simulink model "planta_CODESYS"  (R2025b)
settings: Solver=FixedStepAuto  StartTime=0.0  StopTime=inf  FixedStep=Ts2  MaxStep=1e-3  RelTol=1e-3
undefined symbols (not defined in the file): ah_max, at_max, bcx, bcy, bh_eq, bhb, bhEb, bhwu, bt, bt_eq, btb, btw, g, Hc, ih, it, Jh_eq, Jt_eq, Kcy, khwu, Ki_h, Ki_t, Kp_h, Kp_t, Ktw, lambda, Lh, Lh0, lh_0, Lt, magnitude, Mc_max, Ms, Mt, rhd, rtd, tau_hm, tau_tm, Thb_Max, ThEb_Max, Thm_0, Thm_Max, titahm_0, titatm_0, Ts0, Ts1, Ts2, Ttb_Max, Ttm_0, Ttm_Max, vh_0, vlx_0, vly_0, vt_0, vt_max, Wc, whm_0, whm_rated, wtm_0, xl_0 ... (+9)
libraries: simulink x10, opcualib x9, simulink_extras x2, dspnetwork x2, sl3dlib x1, hostiolib x1
(part 1 of 2)
settings Model: Creator=Nahuel  LastModifiedBy=nahue
settings SolverCC: ZeroCrossControl=DisableAll
settings DebuggingCC: UnderSpecifiedDimensionMsg=warning
settings SFSimCC: SimTargetLang=C++  SimDLTargetLibrary=mkl-dnn
settings RTWCC: GPUComputeCapability=3.5

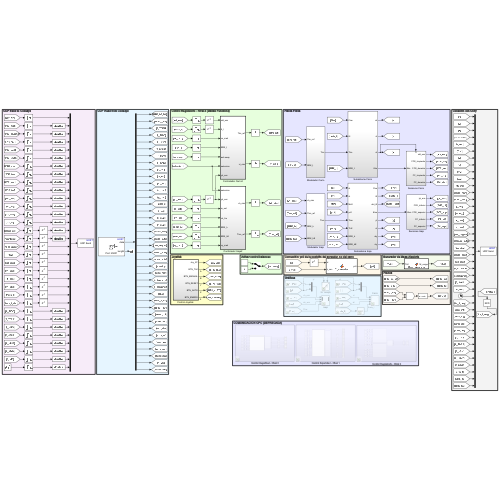
[thumbnail: Simulink's stored preview of the top-level diagram]
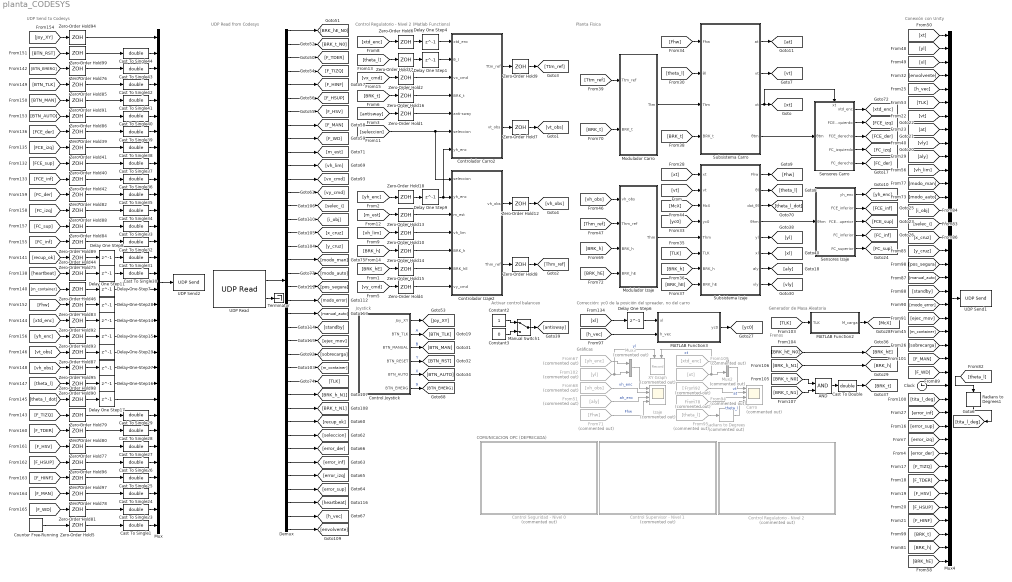
== system planta_CODESYS ==
  note: COMUNICACION OPC (DEPRECADA)
  note: UDP Read from Codesys
  note: UDP Send to Codesys
  note: Joystick
  note: Conexión con Unity
  note: Planta Física
  note: Control Regulatorio - Nivel 2 (Matlab Functions)
  note: Generador de Masa Aleatoria
  note: Corrección: yc0 de la posición del spreader, no del carro
  note: Activar control balanceo
  note: Frenos
  note: Gráficas
  AND : Logic  IconShape=distinctive  AllPortsSameDT=off  OutDataTypeStr=boolean
  Carro : Scope  Commented=on  NumInputPorts=4
      settings: AxesScalingNumUpdates=5  ActiveDisplayYMinimum=-26.90845  ActiveDisplayYMaximum=42.17601
  Cast To Double : DataTypeConversion  OutDataTypeStr=double  SaturateOnIntegerOverflow=off  RndMeth=Floor
  Cast To Single{1,23..44} (23 alike) : DataTypeConversion  OutDataTypeStr=double  SaturateOnIntegerOverflow=off  RndMeth=Floor
  Clock : Clock
  Constant2 : Constant
  Constant3 : Constant  Value=0
  "Control Joystick " : Subsystem  TreatAsAtomicUnit=on  SystemSampleTime=Ts2
  "Control Regulatorio - Nivel 2 " : Subsystem  Commented=on
  Control Seguridad - Nivel 0 : Subsystem  Commented=on
  Control Supervisor - Nivel 1 : Subsystem  Commented=on
  Controlador Carro2 : Subsystem  Priority=3  TreatAsAtomicUnit=on  SystemSampleTime=Ts2
  Controlador Izaje2 : Subsystem  Priority=3  TreatAsAtomicUnit=on  SystemSampleTime=Ts2
  Counter Free-Running : simulink/Sources/Counter Free-Running  NumBits=8  tsamp=Ts1
  Delay One Step{1,7..8,11,16..17,27,29} (8 alike) : Delay  DelayLength=1  InitialCondition=0
  Delay One Step14 : Delay  DelayLength=1  InitialCondition=xt_0
  Delay One Step15 : Delay  DelayLength=1  InitialCondition=yh_0
  Delay One Step28 : Delay  DelayLength=1
  Delay One Step4 : Delay  DelayLength=1  InitialCondition=xtd_0
  Delay One Step6 : Delay  DelayLength=1  InitialCondition=xl_0
  Delay One Step9 : Delay  DelayLength=1  InitialCondition=yh_0
  Demux : Demux  Outputs=[1,1,1,1,1,1,1,1,1, 1,1,1,1, 2, 2, 1,1,1,1,1,1,1,1,1,1,1,1,1,1,1,1,1,1,1,1,1, 33, 33]
  From102 : From  Commented=on  GotoTag=yl
  From109 : From  Commented=on  GotoTag=xtd_enc
  From51 : From  Commented=on  GotoTag=aly
  From67 : From  Commented=on  GotoTag=yh_enc
  From68 : From  Commented=on  GotoTag=vh_obs
  From71 : From  Commented=on  GotoTag=Fhw
  From78 : From  Commented=on  GotoTag=vt_obs
  From92 : From  Commented=on  GotoTag=xt
  From94 : From  Commented=on  GotoTag=at
  From95 : From  Commented=on  GotoTag=theta_l
  Izaje : Scope  Commented=on  NumInputPorts=4
      settings: ActiveDisplayYMinimum=-22.31965  ActiveDisplayYMaximum=45.47272
  MATLAB Function2 : MATLAB Function  TreatAsAtomicUnit=on
  MATLAB Function3 : MATLAB Function  TreatAsAtomicUnit=on
  Manual Switch1 : ManualSwitch
  Modulador Carro : Subsystem
  Modulador Izaje : Subsystem
  Mux : Mux  Inputs=32
  Mux2 : Mux  Commented=on  Inputs=2
  Mux3 : Mux  Commented=on  Inputs=2
  Mux4 : Mux  Inputs=40
  Radians to Degrees : simulink_extras/Transformations/Radians to Degrees  Commented=on
  Radians to Degrees1 : simulink_extras/Transformations/Radians to Degrees
  Sensores Carro : Subsystem
      settings: PortSchema="{\"entries\":[{\"content\":{\"sides\":[{\"content\":{\"connectorIds\":[\"In1\"]},\"type\":\"ConnectorPlacement.EquallySpacedRectSide\",\"uuid\":\"2b8b172e-81b6-42bc-b97d-36a206518a36\"},{\"content\":{\"connectorIds\":[\"Out1\",\"Out2\",\"Out3\",\"Out4\",\"Out5\"],\"side\":\"RIGHT\"},\"type\":\"ConnectorPlacement.EquallySpacedRectSide\",\"uuid\":\"28ef9b2b-04b5-43d8-bbbd-79ec09ba5635\"},{\"content\":{\"connectorIds\":[\"In2\"],\"side\":\"TOP\"},\"type\":\"ConnectorPlacement.EquallySpacedRectSide\",\"uuid\":\"3045eb5d-bca3-4613-a3ba-d9977503ff9f\"}]},\"type\":\"ConnectorPlacement.EquallySpacedConnector\",\"uuid\":\"4bfb3ace-e4bb-48ed-ab64-e99ae27e612e\"}],\"packageUris\":[\"http://schema.mathworks.com/mf0/Connector/R2020b\"],\"version\":\"1.0\"}"
  Sensores Izaje : Subsystem
  Subsistema Carro : Subsystem
  Subsistema Izaje : Subsystem
  Terminator : Terminator
  UDP Read : hostiolib/UDP Read  localURL='0.0.0.0'  localPort=25001  remoteURL='0.0.0.0'  remotePort=-1  recvBufferSize=8192  dims=104  signalDatatype=double  isVarSize=off  showBlockingTime=on  blockingTime=0  sampletime=Ts1  blockPlatform=HOST  hoistedMaskSrc=UDP Read/UDP Read Sim/UDP Read
  UDP Send1 : dspnetwork/UDP Send  remoteURL='127.0.0.1'  remotePort=1234  localURL='0.0.0.0'  localPortSource=Automatically determine  localPort=-1  sendBufferSize=8192  sampletime=-1  blockPlatform=HOST  separateLengthPort=0
  UDP Send2 : dspnetwork/UDP Send  remoteURL='127.0.0.1'  remotePort=25000  localURL='0.0.0.0'  localPortSource=Automatically determine  localPort=-1  sendBufferSize=8192  sampletime=-1  blockPlatform=HOST  separateLengthPort=0
  XY Graph : Record  Commented=on  NumPorts=2.0  FileSettingsInternal="{\"entries\":[{\"content\":{\"excelSettings\":{\"content\":{},\"type\":\"Streamout.ExcelSettings\"},\"parquetSettings\":{\"content\":{},\"type\":\"Streamout.ParquetSettings\"}},\"type\":\"Streamout.FileSettingStorage\",\"uuid\":\"\"}],\"packageUris\":[\"http:\\/\\/schema.mathworks.com\\/mf0\\/streamout_blocks\\/R2020a\"],\"version\":\"1.0\"}"  FrameSettings=[0, 0]  Layout=[1 1]  SignalsInternal="{\"entries\":[{\"content\":{\"signals\":[{\"content\":{\"blockPath\":[],\"dimensions\":[1],\"domain\":\"\",\"lineColor\":\"#a2142f\",\"plots\":[ 1 ],\"port\":1,\"signalID\":1,\"signalName\":\"yl\"},\"type\":\"RecordBlkView.Signal\",\"uuid\":\"\"},{\"content\":{\"blockPath\":[],\"dimensions\":[1],\"domain\":\"\",\"lineColor\":\"#139fff\",\"plots\":[ 1 ],\"port\":2,\"signalID\":2,\"signalName\":\"xt\"},\"type\":\"RecordBlkView.Signal\",\"uuid\":\"\"}]},\"type\":\"RecordBlkView.InputSignals\",\"uuid\":\"\"}],\"packageUris\":[\"http:\\/\\/schema.mathworks.com\\/mf0\\/streamout_blocks\\/R2020a\"],\"version\":\"1.0\"}"  VisualizationBindings="{\"xyplotplugin\":{\"info\":[{\"series\":[{\"bindingParametersList\":[{\"parameter\":\"X-Axis\",\"signalID\":2,\"signalName\":\"xt\"},{\"parameter\":\"Y-Axis\",\"signalID\":1,\"signalName\":\"yl\"}],\"seriesID\":0}],\"subplotID\":1}]}}"  CompatibilityTag=XY
  Zero-Order Hold{1..2,4,6..10,12..16,18,37} (15 alike) : ZeroOrderHold  SampleTime=Ts2
  Zero-Order Hold{5,39..42,44,46,75..76} (9 alike) : ZeroOrderHold  SampleTime=Ts0
  Zero-Order Hold{77..99} (23 alike) : ZeroOrderHold  SampleTime=Ts1
  wires:
  "Control Joystick "/2(BTN_TLK) -> [BTN_TLK]  "A"
  "Control Joystick "/1(Joy_XY) -> [Joy_XY]
  "Control Joystick "/5(BTN_AUTO) -> [BTN_AUTO]  "X"
  "Control Joystick "/4(BTN_RESET) -> [BTN_RST]  "Y"
  "Control Joystick "/3(BTN_MANUAL) -> [BTN_MAN]  "B"
  "Control Joystick "/6(BTN_EMERG) -> [BTN_EMERG]  "9"
  [BRK_h] -> Mux4/39
  Clock/1 -> Mux4/27
  [modo_man] -> Mux4/12
  Mux4/1 -> UDP Send1/1
  [TLK] -> Mux4/6
  [manual_auto] -> Mux4/19
  [F_HSV] -> Mux4/35
  [y_cruz] -> Mux4/17
  Radians to Degrees1/1 -> [tita_l_deg]
  [vt] -> Mux4/7
  [vly] -> Mux4/9
  [modo_error] -> Mux4/21
  [m_container] -> Mux4/23
  [ejec_mov] -> Mux4/22
  [error_der] -> Mux4/32
  [at] -> Mux4/8
  [h_vec] -> Mux4/5
  [F_TIZQ] -> Mux4/33
  [tita_l_deg] -> Mux4/28
  [theta_l] -> Radians to Degrees1/1
  [x_cruz] -> Mux4/16
  [pos_segura] -> Mux4/18
  [BRK_hE] -> Mux4/40
  [error_izq] -> Mux4/31
  [F_MAN] -> Mux4/25
  [selec_i] -> Mux4/15
  [F_WD] -> Mux4/26
  [F_HINF] -> Mux4/37
  [vh_lim] -> Mux4/11
  [error_inf] -> Mux4/29
  [sobrecarga] -> Mux4/24
  [i_obj] -> Mux4/14
  [yl] -> Mux4/2
  [error_sup] -> Mux4/30
  [aly] -> Mux4/10
  [xl] -> Mux4/3
  [F_HSUP] -> Mux4/36
  [modo_auto] -> Mux4/13
  [envolvente] -> Mux4/4
  [F_TDER] -> Mux4/34
  [xt] -> Mux4/1
  [standby] -> Mux4/20
  [BRK_t] -> Mux4/38
  Subsistema Izaje/6(xl) -> [xl]
  Sensores Izaje/5(FC_superior) -> [FC_sup]
  Subsistema Carro/3(xt) -> Sensores Carro/2(xt), [xt]
  Subsistema Izaje/2(θl) -> [theta_l]
  [vt] -> Subsistema Izaje/2(vt)
  Subsistema Carro/4(θtm) -> Sensores Carro/1(θtm)
  Sensores Carro/3(FCE_derecho) -> [FCE_der]
  Sensores Carro/4(FC_izquierdo) -> [FC_izq]
  Modulador Carro/1(Ttm) -> Subsistema Carro/3(Ttm)
  [BRK_hE] -> Modulador Izaje/4(BRK_hE)
  [yc0] -> Subsistema Izaje/4(yc0)
  Subsistema Carro/1(at) -> [at]
  Sensores Carro/2(FCE_izquierdo) -> [FCE_izq]
  [BRK_t] -> Subsistema Carro/4(BRK_t)
  Subsistema Izaje/3(dot_θl) -> [theta_l_dot]
  Sensores Carro/1(xtd_enc) -> [xtd_enc]
  Sensores Izaje/1(yh_enc) -> [yh_enc]
  Modulador Izaje/1(Thm) -> Subsistema Izaje/5(Thm)
  Subsistema Izaje/1(Fhw) -> [Fhw]
  [BRK_h] -> Subsistema Izaje/7(BRK_h)
  Subsistema Izaje/5(yl) -> [yl]
  Sensores Izaje/3(FCE_superior) -> [FCE_sup]
  [Fhw] -> Subsistema Carro/1(Fhw)
  [BRK_hE] -> Subsistema Izaje/8(BRK_hE)
  [TLK] -> Subsistema Izaje/6(TLK)
  [Thm_ref] -> Modulador Izaje/2(Thm_ref)
  [BRK_t] -> Modulador Carro/2(BRK_t)
  Subsistema Izaje/4(θhm) -> Sensores Izaje/1(θhm)
  [xt] -> Subsistema Izaje/1(xt)
  Subsistema Carro/2(vt) -> [vt]
  Sensores Izaje/4(FC_inferior) -> [FC_inf]
  Subsistema Izaje/8(vly) -> [vly]
  Subsistema Izaje/7(aly) -> [aly]
  [BRK_h] -> Modulador Izaje/3(BRK_h)
  Sensores Izaje/2(FCE_inferior) -> [FCE_inf]
  [Ttm_ref] -> Modulador Carro/1(Ttm_ref)
  [McX] -> Subsistema Izaje/3(McX)
  [vh_obs] -> Modulador Izaje/1(vh_obs)
  Sensores Carro/5(FC_derecho) -> [FC_der]
  [theta_l] -> Subsistema Carro/2(θl)
  Zero-Order Hold12/1 -> [vh_obs]
  [seleccion] -> Controlador Carro2/6(seleccion), Controlador Izaje2/1(seleccion)
  [m_est] -> Zero-Order Hold13/1
  Controlador Izaje2/2(Thm_ref) -> Zero-Order Hold8/1
  Delay One Step1/1 -> Controlador Carro2/2(θ_l)
  Controlador Carro2/1(Ttm_ref) -> Zero-Order Hold9/1
  Zero-Order Hold10/1 -> Controlador Izaje2/4(vh_lim)
  [yh_enc] -> Zero-Order Hold18/1
  [BRK_t] -> Zero-Order Hold16/1
  [vh_lim] -> Zero-Order Hold10/1
  Zero-Order Hold7/1 -> [vt_obs]
  [vx_cmd] -> Zero-Order Hold2/1
  [BRK_h] -> Zero-Order Hold14/1
  Delay One Step9/1 -> Controlador Carro2/7(yh_enc), Controlador Izaje2/2(yh_enc)
  Zero-Order Hold16/1 -> Controlador Carro2/4(BRK_t)
  Zero-Order Hold8/1 -> [Thm_ref]
  Delay One Step4/1 -> Controlador Carro2/1(xtd_enc)
  Zero-Order Hold6/1 -> Delay One Step4/1
  Zero-Order Hold2/1 -> Controlador Carro2/3(vx_cmd)
  [theta_l] -> Zero-Order Hold37/1
  Zero-Order Hold37/1 -> Delay One Step1/1
  Zero-Order Hold1/1 -> Controlador Carro2/5(anti-sway)
  Controlador Carro2/2(vt_obs) -> Zero-Order Hold7/1
  [vy_cmd] -> Zero-Order Hold4/1
  Controlador Izaje2/1(vh_obs) -> Zero-Order Hold12/1
  Zero-Order Hold9/1 -> [Ttm_ref]
  Zero-Order Hold18/1 -> Delay One Step9/1
  Zero-Order Hold4/1 -> Controlador Izaje2/7(vy_cmd)
  [antisway] -> Zero-Order Hold1/1
  [xtd_enc] -> Zero-Order Hold6/1
  [BRK_hE] -> Zero-Order Hold15/1
  Zero-Order Hold13/1 -> Controlador Izaje2/3(m_est)
  Zero-Order Hold14/1 -> Controlador Izaje2/5(BRK_h)
  Zero-Order Hold15/1 -> Controlador Izaje2/6(BRK_hE)
  From94/1 -> Carro/3  "at"
  [xl] -> Delay One Step6/1
  [BRK_t_N0] -> AND/1
  Mux2/1 -> Carro/1
  From67/1 -> Mux3/1
  AND/1 -> Cast To Double/1
  Delay One Step6/1 -> MATLAB Function3/1(xl)
  [BRK_t_N1] -> AND/2
  Constant2/1 -> Manual Switch1/1
  MATLAB Function2/1(M_carga) -> [McX]
  From78/1 -> Carro/2  "vt"
  From71/1 -> Izaje/4  "Fhw"
  [h_vec] -> MATLAB Function3/2(h_vec)
  From102/1 -> Mux3/2, XY Graph/1  "yl"
  From92/1 -> Mux2/2, XY Graph/2  "xt"
  Mux3/1 -> Izaje/1
  Cast To Double/1 -> [BRK_t]
  Radians to Degrees/1 -> Carro/4  "theta_l"
  Manual Switch1/1 -> [antisway]
  MATLAB Function3/1(yc0) -> [yc0]
  From68/1 -> Izaje/2  "vh_enc"
  [TLK] -> MATLAB Function2/1(TLK)
  [BRK_h_N1] -> [BRK_h]
  From95/1 -> Radians to Degrees/1
  From51/1 -> Izaje/3  "ah_enc"
  From109/1 -> Mux2/1
  [BRK_hE_N0] -> [BRK_hE]
  Constant3/1 -> Manual Switch1/2
  Zero-Order Hold75/1 -> Delay One Step8/1
  [FCE_sup] -> Zero-Order Hold40/1
  Zero-Order Hold40/1 -> Cast To Single37/1
  Zero-Order Hold41/1 -> Cast To Single38/1
  Zero-Order Hold42/1 -> Cast To Single36/1
  [FCE_der] -> Zero-Order Hold39/1
  [m_container] -> Zero-Order Hold46/1
  [FCE_izq] -> Zero-Order Hold41/1
  Zero-Order Hold76/1 -> Cast To Single43/1
  Zero-Order Hold46/1 -> Delay One Step7/1
  [recup_ok] -> Zero-Order Hold75/1
  Zero-Order Hold39/1 -> Cast To Single39/1
  [BTN_EMERG] -> Zero-Order Hold76/1
  Zero-Order Hold44/1 -> Delay One Step11/1
  [FCE_inf] -> Zero-Order Hold42/1
  [heartbeat] -> Zero-Order Hold44/1
  Delay One Step15/1 -> Mux/20
  Zero-Order Hold80/1 -> Cast To Single28/1
  [F_HSV] -> Zero-Order Hold77/1
  Delay One Step28/1 -> Mux/18
  Zero-Order Hold77/1 -> Cast To Single27/1
  Zero-Order Hold90/1 -> Delay One Step16/1
  [F_HSUP] -> Zero-Order Hold96/1
  Zero-Order Hold79/1 -> Cast To Single29/1
  Zero-Order Hold83/1 -> Delay One Step28/1
  [FC_izq] -> Zero-Order Hold88/1
  [F_MAN] -> Zero-Order Hold78/1
  [vt_obs] -> Zero-Order Hold87/1
  [FC_sup] -> Zero-Order Hold84/1
  [Fhw] -> Zero-Order Hold83/1
  [FC_der] -> Zero-Order Hold82/1
  [theta_l] -> Zero-Order Hold90/1
  Zero-Order Hold97/1 -> Cast To Single25/1
  [F_HINF] -> Zero-Order Hold97/1
  Zero-Order Hold89/1 -> Cast To Single32/1
  Zero-Order Hold94/1 -> Mux/1
  [F_TDER] -> Zero-Order Hold80/1
  Zero-Order Hold88/1 -> Cast To Single34/1
  Zero-Order Hold87/1 -> Delay One Step29/1
  [xtd_enc] -> Zero-Order Hold92/1
  [F_TIZQ] -> Zero-Order Hold79/1
  [Joy_XY] -> Zero-Order Hold94/1
  Zero-Order Hold78/1 -> Cast To Single24/1
  Zero-Order Hold92/1 -> Delay One Step14/1
  Delay One Step14/1 -> Mux/19
  Zero-Order Hold99/1 -> Cast To Single44/1
  Zero-Order Hold82/1 -> Cast To Single35/1
  [theta_l_dot] -> Zero-Order Hold98/1
  Zero-Order Hold98/1 -> Delay One Step17/1
  [BTN_RST] -> Zero-Order Hold99/1
  Zero-Order Hold96/1 -> Cast To Single26/1
  [FC_inf] -> Zero-Order Hold89/1
  Delay One Step17/1 -> Mux/24
  Zero-Order Hold95/1 -> Delay One Step27/1
  Zero-Order Hold84/1 -> Cast To Single33/1
  Delay One Step16/1 -> Mux/23
  Zero-Order Hold93/1 -> Delay One Step15/1
  [F_WD] -> Zero-Order Hold81/1
  [yh_enc] -> Zero-Order Hold93/1
  [vh_obs] -> Zero-Order Hold95/1
  Zero-Order Hold81/1 -> Cast To Single23/1
  Delay One Step29/1 -> Mux/21
  [BTN_TLK] -> Zero-Order Hold85/1
  [BTN_AUTO] -> Zero-Order Hold86/1
  Zero-Order Hold86/1 -> Cast To Single40/1
  Zero-Order Hold91/1 -> Cast To Single41/1
  [BTN_MAN] -> Zero-Order Hold91/1
  Zero-Order Hold85/1 -> Cast To Single42/1
  Delay One Step7/1 -> Mux/17
  Delay One Step11/1 -> Cast To Single30/1
  Delay One Step8/1 -> Cast To Single31/1
  Cast To Single44/1 -> Mux/2
  Cast To Single43/1 -> Mux/3
  Cast To Single42/1 -> Mux/4
  Cast To Single41/1 -> Mux/5
  Cast To Single40/1 -> Mux/6
  Cast To Single39/1 -> Mux/7
  Cast To Single38/1 -> Mux/8
  Cast To Single37/1 -> Mux/9
  Cast To Single36/1 -> Mux/10
  Cast To Single35/1 -> Mux/11
  Cast To Single34/1 -> Mux/12
  Cast To Single33/1 -> Mux/13
  Cast To Single32/1 -> Mux/14
  Cast To Single31/1 -> Mux/15
  Cast To Single30/1 -> Mux/16
  Cast To Single29/1 -> Mux/25
  Cast To Single28/1 -> Mux/26
  Cast To Single27/1 -> Mux/27
  Cast To Single26/1 -> Mux/28
  Cast To Single25/1 -> Mux/29
  Cast To Single24/1 -> Mux/30
  Cast To Single23/1 -> Mux/31
  Delay One Step27/1 -> Mux/22
  UDP Read/2 -> Terminator/1
  UDP Read/1 -> Demux/1
  Demux/35 -> [error_sup]
  Demux/36 -> [heartbeat]
  Demux/37 -> [h_vec]
  Demux/38 -> [envolvente]
  Demux/34 -> [error_izq]
  Demux/33 -> [error_inf]
  Demux/32 -> [error_der]
  Demux/31 -> [seleccion]
  Demux/30 -> [recup_ok]
  Demux/29 -> [BRK_t_N1]
  Demux/28 -> [BRK_h_N1]
  Demux/27 -> [TLK]
  Demux/26 -> [m_container]
  Demux/25 -> [sobrecarga]
  Demux/24 -> [ejec_mov]
  Demux/23 -> [standby]
  Demux/22 -> [manual_auto]
  Demux/21 -> [modo_error]
  Demux/20 -> [pos_segura]
  Demux/19 -> [modo_auto]
  Demux/18 -> [modo_man]
  Demux/17 -> [y_cruz]
  Demux/16 -> [x_cruz]
  Demux/15 -> [i_obj]
  Demux/14 -> [selec_i]
  Demux/13 -> [vy_cmd]
  Demux/11 -> [vh_lim]
  Demux/12 -> [vx_cmd]
  Demux/10 -> [m_est]
  Demux/9 -> [F_WD]
  Demux/8 -> [F_MAN]
  Demux/7 -> [F_HSV]
  Demux/6 -> [F_HSUP]
  Demux/5 -> [F_HINF]
  Demux/4 -> [F_TIZQ]
  Demux/3 -> [F_TDER]
  Demux/2 -> [BRK_t_N0]
  Demux/1 -> [BRK_hE_N0]
  Counter Free-Running/1 -> Zero-Order Hold5/1
  Cast To Single1/1 -> Mux/32
  Mux/1 -> UDP Send2/1
  Zero-Order Hold5/1 -> Cast To Single1/1

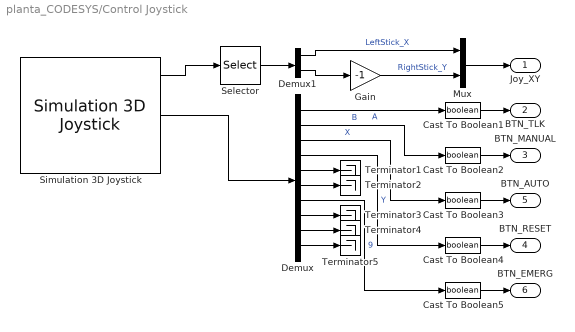
== system planta_CODESYS/Control Joystick  ==
  Cast To Boolean{1..5} (5 alike) : DataTypeConversion  OutDataTypeStr=boolean  SaturateOnIntegerOverflow=off  RndMeth=Floor
  Demux : Demux  Outputs=10
  Demux1 : Demux  Outputs=2
  Gain : Gain  Gain=-1
  Mux : Mux  Inputs=2
  Selector : Selector  InputPortWidth=5  IndexOptions=Index vector (dialog)  Indices=[1 5]  OutputSizes=1
  Simulation 3D Joystick : sl3dlib/Simulation 3D/Hardware Interface/Simulation 3D Joystick  joyid=1  adjustports=on  forcefeed=off
  Terminator{1..5} (5 alike) : Terminator
  Joy_XY : Outport
  BTN_TLK : Outport  Port=2
  BTN_MANUAL : Outport  Port=3
  BTN_RESET : Outport  Port=4
  BTN_AUTO : Outport  Port=5
  BTN_EMERG : Outport  Port=6
  wires:
  Demux/1 -> Cast To Boolean1/1  "A"
  Demux1/2 -> Gain/1
  Demux1/1 -> Mux/1  "LeftStick_X"
  Selector/1 -> Demux1/1
  Simulation 3D Joystick/1 -> Selector/1
  Gain/1 -> Mux/2  "RightStick_Y"
  Simulation 3D Joystick/2 -> Demux/1
  Demux/2 -> Cast To Boolean2/1  "B"
  Demux/3 -> Cast To Boolean3/1  "X"
  Demux/4 -> Cast To Boolean4/1  "Y"
  Mux/1 -> Joy_XY/1
  Demux/5 -> Terminator1/1
  Demux/6 -> Terminator2/1
  Demux/8 -> Terminator3/1
  Demux/9 -> Terminator4/1
  Demux/10 -> Terminator5/1
  Demux/7 -> Cast To Boolean5/1  "9"
  Cast To Boolean1/1 -> BTN_TLK/1
  Cast To Boolean2/1 -> BTN_MANUAL/1
  Cast To Boolean3/1 -> BTN_AUTO/1
  Cast To Boolean4/1 -> BTN_RESET/1
  Cast To Boolean5/1 -> BTN_EMERG/1

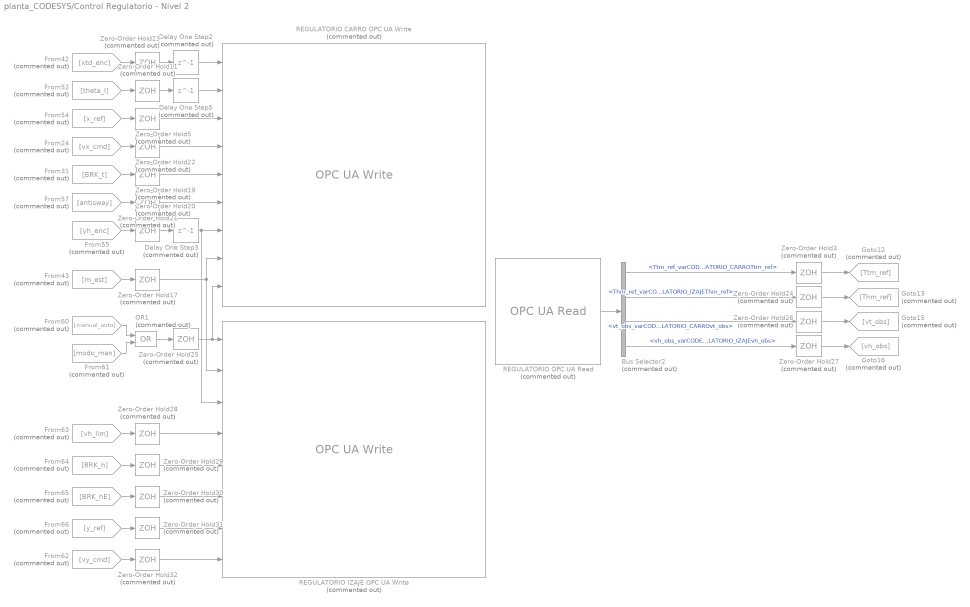
== system planta_CODESYS/Control Regulatorio - Nivel 2  ==
  Bus Selector2 : BusSelector  Commented=on  OutputSignals=Ttm_ref_varCODESYSControlWinV3X64CONTROL_REGULATORIO_CARROTtm_ref,Thm_ref_varCODESYSControlWinV3X64CONTROL_REGULATORIO_IZAJEThm_ref,vt_obs_varCODESYSControlWinV3X64CONTROL_REGULATORIO_CARROvt_obs,vh_obs_varCODESYSControlWinV3X64CONTROL_REGULATORIO_IZAJEvh_obs
  Delay One Step2 : Delay  Commented=on  DelayLength=1  InitialCondition=xtd_0
  Delay One Step3 : Delay  Commented=on  DelayLength=1  InitialCondition=yh_0
  Delay One Step5 : Delay  Commented=on  DelayLength=1  InitialCondition=0
  From24 : From  Commented=on  GotoTag=vx_cmd
  From31 : From  Commented=on  GotoTag=BRK_t
  From42 : From  Commented=on  GotoTag=xtd_enc
  From43 : From  Commented=on  GotoTag=m_est
  From52 : From  Commented=on  GotoTag=theta_l
  From54 : From  Commented=on  GotoTag=x_ref
  From55 : From  Commented=on  GotoTag=yh_enc
  From57 : From  Commented=on  GotoTag=antisway
  From60 : From  Commented=on  GotoTag=manual_auto
  From61 : From  Commented=on  GotoTag=modo_man
  From62 : From  Commented=on  GotoTag=vy_cmd
  From63 : From  Commented=on  GotoTag=vh_lim
  From64 : From  Commented=on  GotoTag=BRK_h
  From65 : From  Commented=on  GotoTag=BRK_hE
  From66 : From  Commented=on  GotoTag=y_ref
  Goto12 : Goto  Commented=on  GotoTag=Ttm_ref
  Goto13 : Goto  Commented=on  GotoTag=Thm_ref
  Goto15 : Goto  Commented=on  GotoTag=vt_obs
  Goto16 : Goto  Commented=on  GotoTag=vh_obs
  OR1 : Logic  Commented=on  Operator=OR  IconShape=distinctive  AllPortsSameDT=off  OutDataTypeStr=boolean
  REGULATORIO CARRO OPC UA Write : opcualib/OPC UA Write  Commented=on  SelectedServer=OPCUAServer@LEGION-Rodri  ServerList=OPCUAServer@LEGION-Rodri  SampleTime=0.1  NodeList={ '1', 'xtd_enc', '4', '|var|CODESYS Control Win V3 x64.CONTROL_REGULATORIO_CARRO.xtd_enc', '0'; '2', 'tita_l', '4', '|var|CODESYS Control Win V3 x64.CONTROL_REGULATORIO_CARRO.tita_l', '0'; '3', 'xt_ref', '4', '|var|CODESYS Control Win V3 x64.CONTROL_REGULATORIO_CARRO.xt_ref', '0'; '4', 'vx_cmd', '4', '|var|CODESYS Control Win V3 x64.CONTROL_REGULATORIO_CARRO.vx_cmd', '0'; '5', 'BRK_t', '4', '|var|CODESYS Control Win V3 x64.CONTROL_REGULATORIO_CARRO.BRK_t', '0'; '6', 'antisway', '4', '|var|CODESYS Control Win V3 x64.CONTROL_REGULATORIO_CARRO.antisway', '0'; '7', 'yh_enc', '4', '|var|CODESYS Control Win V3 x64.CONTROL_REGULATORIO_CARRO.yh_enc', '0'; '8', 'm_est', '4', '|var|CODESYS Control Win V3 x64.CONTROL_REGULATORIO_CARRO.m_est', '0'; '9', 'modo_manual', '4', '|var|CODESYS Control Win V3 x64.CONTROL_REGULATORIO_CARRO.modo_manual', '0' }
  REGULATORIO IZAJE OPC UA Write : opcualib/OPC UA Write  Commented=on  SelectedServer=OPCUAServer@LEGION-Rodri  ServerList=OPCUAServer@LEGION-Rodri  SampleTime=0.1  NodeList={ '1', 'modo_manual', '4', '|var|CODESYS Control Win V3 x64.CONTROL_REGULATORIO_IZAJE.modo_manual', '0'; '2', 'm_est', '4', '|var|CODESYS Control Win V3 x64.CONTROL_REGULATORIO_IZAJE.m_est', '0'; '3', 'yh_enc', '4', '|var|CODESYS Control Win V3 x64.CONTROL_REGULATORIO_IZAJE.yh_enc', '0'; '4', 'vh_lim', '4', '|var|CODESYS Control Win V3 x64.CONTROL_REGULATORIO_IZAJE.vh_lim', '0'; '5', 'BRK_h', '4', '|var|CODESYS Control Win V3 x64.CONTROL_REGULATORIO_IZAJE.BRK_h', '0'; '6', 'BRK_hE', '4', '|var|CODESYS Control Win V3 x64.CONTROL_REGULATORIO_IZAJE.BRK_hE', '0'; '7', 'yh_ref', '4', '|var|CODESYS Control Win V3 x64.CONTROL_REGULATORIO_IZAJE.yh_ref', '0'; '8', 'vy_cmd', '4', '|var|CODESYS Control Win V3 x64.CONTROL_REGULATORIO_IZAJE.vy_cmd', '0' }
  REGULATORIO OPC UA Read : opcualib/OPC UA Read  Commented=on  SelectedServer=OPCUAServer@LEGION-Rodri  ServerList=OPCUAServer@LEGION-Rodri  NodeList={ '1', 'Ttm_ref', '4', '|var|CODESYS Control Win V3 x64.CONTROL_REGULATORIO_CARRO.Ttm_ref', '0'; '2', 'Thm_ref', '4', '|var|CODESYS Control Win V3 x64.CONTROL_REGULATORIO_IZAJE.Thm_ref', '0'; '3', 'vt_obs', '4', '|var|CODESYS Control Win V3 x64.CONTROL_REGULATORIO_CARRO.vt_obs', '0'; '4', 'vh_obs', '4', '|var|CODESYS Control Win V3 x64.CONTROL_REGULATORIO_IZAJE.vh_obs', '0' }  ShowQualityPort=off  ShowTimestampPort=off  ShowTimestampPortAs=Seconds since start  SampleTime=0.1
  Zero-Order Hold{3,5,11,17,19..32} (18 alike) : ZeroOrderHold  Commented=on  SampleTime=Ts2
  wires:
  From64/1 -> Zero-Order Hold29/1
  Zero-Order Hold21/1 -> REGULATORIO CARRO OPC UA Write/6
  Zero-Order Hold17/1 -> REGULATORIO IZAJE OPC UA Write/2, REGULATORIO CARRO OPC UA Write/8
  From61/1 -> OR1/2
  Zero-Order Hold32/1 -> REGULATORIO IZAJE OPC UA Write/8
  From42/1 -> Zero-Order Hold23/1
  REGULATORIO OPC UA Read/1 -> Bus Selector2/1
  Zero-Order Hold19/1 -> REGULATORIO CARRO OPC UA Write/5
  Delay One Step3/1 -> REGULATORIO IZAJE OPC UA Write/3, REGULATORIO CARRO OPC UA Write/7
  From57/1 -> Zero-Order Hold21/1
  Zero-Order Hold28/1 -> REGULATORIO IZAJE OPC UA Write/4
  From43/1 -> Zero-Order Hold17/1
  Zero-Order Hold29/1 -> REGULATORIO IZAJE OPC UA Write/5
  From31/1 -> Zero-Order Hold19/1
  From65/1 -> Zero-Order Hold30/1
  Zero-Order Hold22/1 -> REGULATORIO CARRO OPC UA Write/4
  Delay One Step5/1 -> REGULATORIO CARRO OPC UA Write/2
  From66/1 -> Zero-Order Hold31/1
  Zero-Order Hold24/1 -> Goto13/1
  Bus Selector2/2 -> Zero-Order Hold24/1  "<Thm_ref_varCODESYSControlWinV3X64CONTROL_REGULATORIO_IZAJEThm_ref>"
  Bus Selector2/3 -> Zero-Order Hold26/1  "<vt_obs_varCODESYSControlWinV3X64CONTROL_REGULATORIO_CARROvt_obs>"
  From60/1 -> OR1/1
  From54/1 -> Zero-Order Hold5/1
  From24/1 -> Zero-Order Hold22/1
  From63/1 -> Zero-Order Hold28/1
  Zero-Order Hold23/1 -> Delay One Step2/1
  Delay One Step2/1 -> REGULATORIO CARRO OPC UA Write/1
  Zero-Order Hold27/1 -> Goto16/1
  Bus Selector2/1 -> Zero-Order Hold3/1  "<Ttm_ref_varCODESYSControlWinV3X64CONTROL_REGULATORIO_CARROTtm_ref>"
  Zero-Order Hold20/1 -> Delay One Step3/1
  OR1/1 -> Zero-Order Hold25/1
  Zero-Order Hold25/1 -> REGULATORIO CARRO OPC UA Write/9, REGULATORIO IZAJE OPC UA Write/1
  From52/1 -> Zero-Order Hold11/1
  From62/1 -> Zero-Order Hold32/1
  Bus Selector2/4 -> Zero-Order Hold27/1  "<vh_obs_varCODESYSControlWinV3X64CONTROL_REGULATORIO_IZAJEvh_obs>"
  Zero-Order Hold5/1 -> REGULATORIO CARRO OPC UA Write/3
  Zero-Order Hold11/1 -> Delay One Step5/1
  Zero-Order Hold30/1 -> REGULATORIO IZAJE OPC UA Write/6
  Zero-Order Hold31/1 -> REGULATORIO IZAJE OPC UA Write/7
  Zero-Order Hold3/1 -> Goto12/1
  From55/1 -> Zero-Order Hold20/1
  Zero-Order Hold26/1 -> Goto15/1

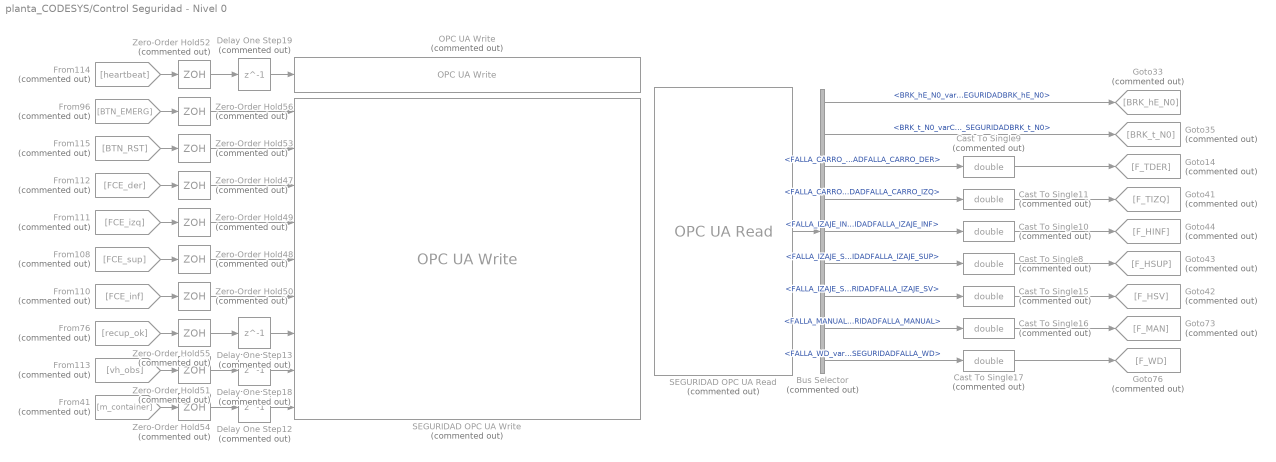
== system planta_CODESYS/Control Seguridad - Nivel 0 ==
  Bus Selector : BusSelector  Commented=on  OutputSignals=BRK_hE_N0_varCODESYSControlWinV3X64CONTROL_SEGURIDADBRK_hE_N0,BRK_t_N0_varCODESYSControlWinV3X64CONTROL_SEGURIDADBRK_t_N0,FALLA_CARRO_DER_varCODESYSControlWinV3X64CONTROL_SEGURIDADFALLA_CARRO_DER,FALLA_CARRO_IZQ_varCODESYSControlWinV3X64CONTROL_SEGURIDADFALLA_CARRO_IZQ,FALLA_IZAJE_INF_varCODESYSControlWinV3X64CONTROL_SEGURIDADFALLA_IZAJE_INF,FALLA_IZAJE_SUP_varCODESYSControlWinV3X64CONTROL_SEGURIDADFALLA_IZAJE_SUP,FALLA_IZAJE_SV_varCODESYSControlWinV3X64CONTROL_SEGURIDADFALLA_IZAJE_SV,FALLA_MANUAL_varCODESYSControlWinV3X64CONTROL_SEGURIDADFALLA_MANUAL,FALLA_WD_varCODESYSControlWinV3X64CONTROL_SEGURIDADFALLA_WD
  Cast To Single{8..11,15..17} (7 alike) : DataTypeConversion  Commented=on  OutDataTypeStr=double  SaturateOnIntegerOverflow=off  RndMeth=Floor
  Delay One Step{12..13,18..19} (4 alike) : Delay  Commented=on  DelayLength=1  InitialCondition=0
  From108 : From  Commented=on  GotoTag=FCE_sup
  From110 : From  Commented=on  GotoTag=FCE_inf
  From111 : From  Commented=on  GotoTag=FCE_izq
  From112 : From  Commented=on  GotoTag=FCE_der
  From113 : From  Commented=on  GotoTag=vh_obs
  From114 : From  Commented=on  GotoTag=heartbeat
  From115 : From  Commented=on  GotoTag=BTN_RST
  From41 : From  Commented=on  GotoTag=m_container
  From76 : From  Commented=on  GotoTag=recup_ok
  From96 : From  Commented=on  GotoTag=BTN_EMERG
  Goto14 : Goto  Commented=on  GotoTag=F_TDER
  Goto33 : Goto  Commented=on  GotoTag=BRK_hE_N0
  Goto35 : Goto  Commented=on  GotoTag=BRK_t_N0
  Goto41 : Goto  Commented=on  GotoTag=F_TIZQ
  Goto42 : Goto  Commented=on  GotoTag=F_HSV
  Goto43 : Goto  Commented=on  GotoTag=F_HSUP
  Goto44 : Goto  Commented=on  GotoTag=F_HINF
  Goto73 : Goto  Commented=on  GotoTag=F_MAN
  Goto76 : Goto  Commented=on  GotoTag=F_WD
  OPC UA Write : opcualib/OPC UA Write  Commented=on  SelectedServer=OPCUAServer@Nahuel  ServerList=OPCUAServer@Nahuel  SampleTime=Ts0  NodeList={ '1', 'heartbeat', '4', '|var|CODESYS Control Win V3 x64.CONTROL_SEGURIDAD.heartbeat', '0' }
  SEGURIDAD OPC UA Read : opcualib/OPC UA Read  Commented=on  SelectedServer=OPCUAServer@Nahuel  ServerList=OPCUAServer@Nahuel  NodeList={ '1', 'BRK_hE_N0', '4', '|var|CODESYS Control Win V3 x64.CONTROL_SEGURIDAD.BRK_hE_N0', '0'; '2', 'BRK_t_N0', '4', '|var|CODESYS Control Win V3 x64.CONTROL_SEGURIDAD.BRK_t_N0', '0'; '3', 'FALLA_CARRO_DER', '4', '|var|CODESYS Control Win V3 x64.CONTROL_SEGURIDAD.FALLA_CARRO_DER', '0'; '4', 'FALLA_CARRO_IZQ', '4', '|var|CODESYS Control Win V3 x64.CONTROL_SEGURIDAD.FALLA_CARRO_IZQ', '0'; '5', 'FALLA_IZAJE_INF', '4', '|var|CODESYS Control Win V3 x64.CONTROL_SEGURIDAD.FALLA_IZAJE_INF', '0'; '6', 'FALLA_IZAJE_SUP', '4', '|var|CODESYS Control Win V3 x64.CONTROL_SEGURIDAD.FALLA_IZAJE_SUP', '0'; '7', 'FALLA_IZAJE_SV', '4', '|var|CODESYS Control Win V3 x64.CONTROL_SEGURIDAD.FALLA_IZAJE_SV', '0'; '8', 'FALLA_MANUAL', '4', '|var|CODESYS Control Win V3 x64.CONTROL_SEGURIDAD.FALLA_MANUAL', '0'; '9', 'FALLA_WD', '4', '|var|CODESYS Control Win V3 x64.CONTROL_SEGURIDAD.FALLA_WD', '0' }  ShowQualityPort=off  ShowTimestampPort=off  ShowTimestampPortAs=Seconds since start  SampleTime=0.5
  SEGURIDAD OPC UA Write : opcualib/OPC UA Write  Commented=on  SelectedServer=OPCUAServer@Nahuel  ServerList=OPCUAServer@Nahuel  SampleTime=0.5  NodeList={ '1', 'BTN_Emerg', '4', '|var|CODESYS Control Win V3 x64.CONTROL_SEGURIDAD.BTN_Emerg', '0'; '2', 'BTN_Reset', '4', '|var|CODESYS Control Win V3 x64.CONTROL_SEGURIDAD.BTN_Reset', '0'; '3', 'FCE_der', '4', '|var|CODESYS Control Win V3 x64.CONTROL_SEGURIDAD.FCE_der', '0'; '4', 'FCE_izq', '4', '|var|CODESYS Control Win V3 x64.CONTROL_SEGURIDAD.FCE_izq', '0'; '5', 'FCE_sup', '4', '|var|CODESYS Control Win V3 x64.CONTROL_SEGURIDAD.FCE_sup', '0'; '6', 'FCE_inf', '4', '|var|CODESYS Control Win V3 x64.CONTROL_SEGURIDAD.FCE_inf', '0'; '7', 'recup_ok', '4', '|var|CODESYS Control Win V3 x64.CONTROL_SEGURIDAD.recup_ok', '0'; '8', 'vh_obs', '4', '|var|CODESYS Control Win V3 x64.CONTROL_SEGURIDAD.vh_obs', '0'; '9', 'm_container', '4', '|var|CODESYS Control Win V3 x64.CONTROL_SEGURIDAD.m_container', '0' }
  Zero-Order Hold{47..56} (10 alike) : ZeroOrderHold  Commented=on  SampleTime=Ts0
  wires:
  From76/1 -> Zero-Order Hold55/1
  Cast To Single10/1 -> Goto44/1
  Bus Selector/6 -> Cast To Single8/1  "<FALLA_IZAJE_SUP_varCODESYSControlWinV3X64CONTROL_SEGURIDADFALLA_IZAJE_SUP>"
  Cast To Single15/1 -> Goto42/1
  From114/1 -> Zero-Order Hold52/1
  Cast To Single16/1 -> Goto73/1
  Bus Selector/9 -> Cast To Single17/1  "<FALLA_WD_varCODESYSControlWinV3X64CONTROL_SEGURIDADFALLA_WD>"
  Bus Selector/4 -> Cast To Single11/1  "<FALLA_CARRO_IZQ_varCODESYSControlWinV3X64CONTROL_SEGURIDADFALLA_CARRO_IZQ>"
  From110/1 -> Zero-Order Hold50/1
  Zero-Order Hold52/1 -> Delay One Step19/1
  From96/1 -> Zero-Order Hold56/1
  Zero-Order Hold47/1 -> SEGURIDAD OPC UA Write/3
  Bus Selector/2 -> Goto35/1  "<BRK_t_N0_varCODESYSControlWinV3X64CONTROL_SEGURIDADBRK_t_N0>"
  Zero-Order Hold54/1 -> Delay One Step12/1
  From115/1 -> Zero-Order Hold53/1
  Bus Selector/7 -> Cast To Single15/1  "<FALLA_IZAJE_SV_varCODESYSControlWinV3X64CONTROL_SEGURIDADFALLA_IZAJE_SV>"
  Zero-Order Hold53/1 -> SEGURIDAD OPC UA Write/2
  Zero-Order Hold50/1 -> SEGURIDAD OPC UA Write/6
  Cast To Single11/1 -> Goto41/1
  Cast To Single8/1 -> Goto43/1
  From112/1 -> Zero-Order Hold47/1
  From108/1 -> Zero-Order Hold48/1
  Bus Selector/5 -> Cast To Single10/1  "<FALLA_IZAJE_INF_varCODESYSControlWinV3X64CONTROL_SEGURIDADFALLA_IZAJE_INF>"
  Zero-Order Hold49/1 -> SEGURIDAD OPC UA Write/4
  Bus Selector/3 -> Cast To Single9/1  "<FALLA_CARRO_DER_varCODESYSControlWinV3X64CONTROL_SEGURIDADFALLA_CARRO_DER>"
  Bus Selector/1 -> Goto33/1  "<BRK_hE_N0_varCODESYSControlWinV3X64CONTROL_SEGURIDADBRK_hE_N0>"
  Zero-Order Hold56/1 -> SEGURIDAD OPC UA Write/1
  Zero-Order Hold51/1 -> Delay One Step18/1
  Zero-Order Hold48/1 -> SEGURIDAD OPC UA Write/5
  From111/1 -> Zero-Order Hold49/1
  Delay One Step19/1 -> OPC UA Write/1
  SEGURIDAD OPC UA Read/1 -> Bus Selector/1
  Cast To Single17/1 -> Goto76/1
  Delay One Step12/1 -> SEGURIDAD OPC UA Write/9
  From41/1 -> Zero-Order Hold54/1
  From113/1 -> Zero-Order Hold51/1
  Cast To Single9/1 -> Goto14/1
  Delay One Step18/1 -> SEGURIDAD OPC UA Write/8
  Bus Selector/8 -> Cast To Single16/1  "<FALLA_MANUAL_varCODESYSControlWinV3X64CONTROL_SEGURIDADFALLA_MANUAL>"
  Zero-Order Hold55/1 -> Delay One Step13/1
  Delay One Step13/1 -> SEGURIDAD OPC UA Write/7

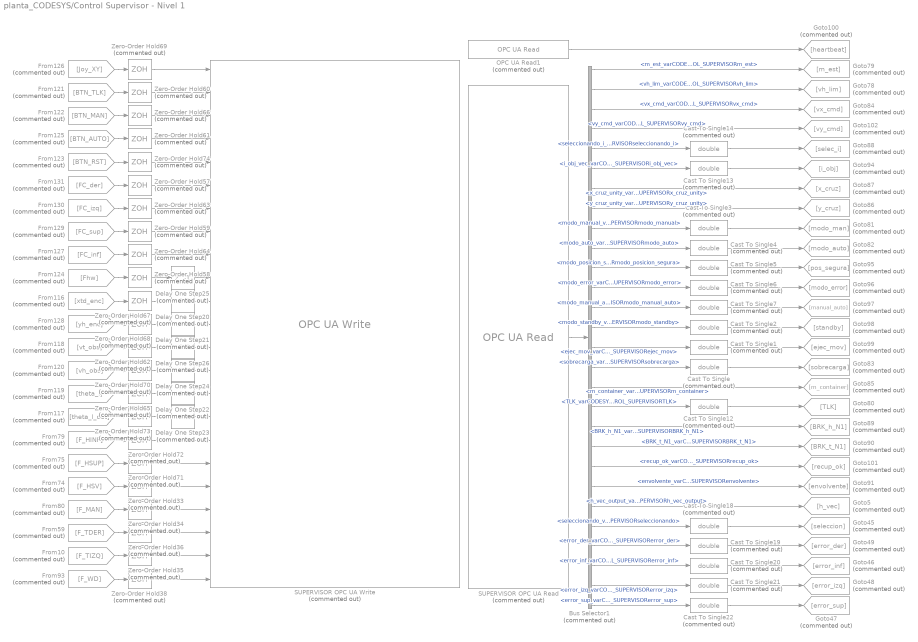
== system planta_CODESYS/Control Supervisor - Nivel 1 ==
  Bus Selector1 : BusSelector  Commented=on  OutputSignals=m_est_varCODESYSControlWinV3X64CONTROL_SUPERVISORm_est,vh_lim_varCODESYSControlWinV3X64CONTROL_SUPERVISORvh_lim,vx_cmd_varCODESYSControlWinV3X64CONTROL_SUPERVISORvx_cmd,vy_cmd_varCODESYSControlWinV3X64CONTROL_SUPERVISORvy_cmd,seleccionando_i_varCODESYSControlWinV3X64CONTROL_SUPERVISORseleccionando_i,i_obj_vec_varCODESYSControlWinV3X64CONTROL_SUPERVISORi_obj_vec,x_cruz_unity_varCODESYSControlWinV3X64CONTROL_SUPERVISORx_cruz_unity,y_cruz_unity_varCODESYSControlWinV3X64CONTROL_SUPERVISORy_cruz_unity,modo_manual_varCODESYSControlWinV3X64CONTROL_SUPERVISORmodo_manual,modo_auto_varCODESYSControlWinV3X64CONTROL_SUPERVISORmodo_auto,modo_posicion_segura_varCODESYSControlWinV3X64CONTROL_SUPERVISORmodo_posicion_segura,modo_error_varCODESYSControlWinV3X64CONTROL_SUPERVISORmodo_error,modo_manual_auto_varCODESYSControlWinV3X64CONTROL_SUPERVISORmodo_manual_auto,modo_standby_varCODESYSControlWinV3X64CONTROL_SUPERVISORmodo_standby,ejec_mov_varCODESYSControlWinV3X64CONTROL_SUPERVISORejec_mov,sobrecarga_varCODESYSControlWinV3X64CONTROL_SUPERVISORsobrecarga,m_container_varCODESYSControlWinV3X64CONTROL_SUPERVISORm_container,TLK_varCODESYSControlWinV3X64CONTROL_SUPERVISORTLK,BRK_h_N1_varCODESYSControlWinV3X64CONTROL_SUPERVISORBRK_h_N1,BRK_t_N1_varCODESYSControlWinV3X64CONTROL_SUPERVISORBRK_t_N1,recup_ok_varCODESYSControlWinV3X64CONTROL_SUPERVISORrecup_ok,envolvente_varCODESYSControlWinV3X64CONTROL_SUPERVISORenvolvente,h_vec_output_varCODESYSControlWinV3X64CONTROL_SUPERVISORh_vec_output,seleccionando_varCODESYSControlWinV3X64CONTROL_SUPERVISORseleccionando,error_der_varCODESYSControlWinV3X64CONTROL_SUPERVISORerror_der,error_inf_varCODESYSControlWinV3X64CONTROL_SUPERVISORerror_inf,error_izq_varCODESYSControlWinV3X64CONTROL_SUPERVISORerror_izq,error_sup_varCODESYSControlWinV3X64CONTROL_SUPERVISORerror_sup
  Cast To Single{,1..7,12..14,18..22} (16 alike) : DataTypeConversion  Commented=on  OutDataTypeStr=double  SaturateOnIntegerOverflow=off  RndMeth=Floor
  Delay One Step20 : Delay  Commented=on  DelayLength=1  InitialCondition=xt_0
  Delay One Step21 : Delay  Commented=on  DelayLength=1  InitialCondition=yh_0
  Delay One Step{22..24,26} (4 alike) : Delay  Commented=on  DelayLength=1  InitialCondition=0
  Delay One Step25 : Delay  Commented=on  DelayLength=1
  From10 : From  Commented=on  GotoTag=F_TIZQ
  From116 : From  Commented=on  GotoTag=xtd_enc
  From117 : From  Commented=on  GotoTag=theta_l_dot
  From118 : From  Commented=on  GotoTag=vt_obs
  From119 : From  Commented=on  GotoTag=theta_l
  From120 : From  Commented=on  GotoTag=vh_obs
  From121 : From  Commented=on  GotoTag=BTN_TLK
  From122 : From  Commented=on  GotoTag=BTN_MAN
  From123 : From  Commented=on  GotoTag=BTN_RST
  From124 : From  Commented=on  GotoTag=Fhw
  From125 : From  Commented=on  GotoTag=BTN_AUTO
  From126 : From  Commented=on  GotoTag=Joy_XY
  From127 : From  Commented=on  GotoTag=FC_inf
  From128 : From  Commented=on  GotoTag=yh_enc
  From129 : From  Commented=on  GotoTag=FC_sup
  From130 : From  Commented=on  GotoTag=FC_izq
  From131 : From  Commented=on  GotoTag=FC_der
  From59 : From  Commented=on  GotoTag=F_TDER
  From74 : From  Commented=on  GotoTag=F_HSV
  From75 : From  Commented=on  GotoTag=F_HSUP
  From79 : From  Commented=on  GotoTag=F_HINF
  From80 : From  Commented=on  GotoTag=F_MAN
  From93 : From  Commented=on  GotoTag=F_WD
  Goto100 : Goto  Commented=on  GotoTag=heartbeat
  Goto101 : Goto  Commented=on  GotoTag=recup_ok
  Goto102 : Goto  Commented=on  GotoTag=vy_cmd
  Goto45 : Goto  Commented=on  GotoTag=seleccion
  Goto46 : Goto  Commented=on  GotoTag=error_inf
  Goto47 : Goto  Commented=on  GotoTag=error_sup
  Goto48 : Goto  Commented=on  GotoTag=error_izq
  Goto49 : Goto  Commented=on  GotoTag=error_der
  Goto5 : Goto  Commented=on  GotoTag=h_vec
  Goto78 : Goto  Commented=on  GotoTag=vh_lim
  Goto79 : Goto  Commented=on  GotoTag=m_est
  Goto80 : Goto  Commented=on  GotoTag=TLK
  Goto81 : Goto  Commented=on  GotoTag=modo_man
  Goto82 : Goto  Commented=on  GotoTag=modo_auto
  Goto83 : Goto  Commented=on  GotoTag=sobrecarga
  Goto84 : Goto  Commented=on  GotoTag=vx_cmd
  Goto85 : Goto  Commented=on  GotoTag=m_container
  Goto86 : Goto  Commented=on  GotoTag=y_cruz
  Goto87 : Goto  Commented=on  GotoTag=x_cruz
  Goto88 : Goto  Commented=on  GotoTag=selec_i
  Goto89 : Goto  Commented=on  GotoTag=BRK_h_N1
  Goto90 : Goto  Commented=on  GotoTag=BRK_t_N1
  Goto91 : Goto  Commented=on  GotoTag=envolvente
  Goto94 : Goto  Commented=on  GotoTag=i_obj
  Goto95 : Goto  Commented=on  GotoTag=pos_segura
  Goto96 : Goto  Commented=on  GotoTag=modo_error
  Goto97 : Goto  Commented=on  GotoTag=manual_auto
  Goto98 : Goto  Commented=on  GotoTag=standby
  Goto99 : Goto  Commented=on  GotoTag=ejec_mov
  OPC UA Read1 : opcualib/OPC UA Read  Commented=on  SelectedServer=OPCUAServer@Nahuel  ServerList=OPCUAServer@Nahuel  NodeList={ '1', 'heartbeat', '4', '|var|CODESYS Control Win V3 x64.CONTROL_SUPERVISOR.heartbeat', '0' }  ShowQualityPort=off  ShowTimestampPort=off  ShowTimestampPortAs=Seconds since start  SampleTime=Ts1
  SUPERVISOR OPC UA Read : opcualib/OPC UA Read  Commented=on  SelectedServer=OPCUAServer@Nahuel  ServerList=OPCUAServer@Nahuel  NodeList={ '1', 'm_est', '4', '|var|CODESYS Control Win V3 x64.CONTROL_SUPERVISOR.m_est', '0'; '2', 'vh_lim', '4', '|var|CODESYS Control Win V3 x64.CONTROL_SUPERVISOR.vh_lim', '0'; '3', 'vx_cmd', '4', '|var|CODESYS Control Win V3 x64.CONTROL_SUPERVISOR.vx_cmd', '0'; '4', 'vy_cmd', '4', '|var|CODESYS Control Win V3 x64.CONTROL_SUPERVISOR.vy_cmd', '0'; '5', 'seleccionando_i', '4', '|var|CODESYS Control Win V3 x64.CONTROL_SUPERVISOR.seleccionando_i', '0'; '6', 'i_obj_vec', '4', '|var|CODESYS Control Win V3 x64.CONTROL_SUPERVISOR.i_obj_vec', '0'; '7', 'x_cruz_unity', '4', '|var|CODESYS Control Win V3 x64.CONTROL_SUPERVISOR.x_cruz_unity', '0'; '8', 'y_cruz_unity', '4', '|var|CODESYS Control Win V3 x64.CONTROL_SUPERVISOR.y_cruz_unity', '0'; '9', 'modo_manual', '4', '|var|CODESYS Control Win V3 x64.CONTROL_SUPERVISOR.modo_manual', '0'; '10', 'modo_auto', '4', '|var|CODESYS Control Win V3 x64.CONTROL_SUPERVISOR.modo_auto', '0'; '11', 'modo_posicion_segura', '4', '|var|CODESYS Control Win V3 x64.CONTROL_SUPERVISOR.modo_posicion_segura', '0'; '12', 'modo_error', '4', '|var|CODESYS Control Win V3 x64.CONTROL_SUPERVISOR.modo_error', '0'; '13', 'modo_manual_auto', '4', '|var|CODESYS Control Win V3 x64.CONTROL_SUPERVISOR.modo_manual_auto', '0'; '14', 'modo_standby', '4', '|var|CODESYS Control Win V3 x64.CONTROL_SUPERVISOR.modo_standby', '0'; '15', 'ejec_mov', '4', '|var|CODESYS Control Win V3 x64.CONTROL_SUPERVISOR.ejec_mov', '0'; '16', 'sobrecarga', '4', '|var|CODESYS Control Win V3 x64.CONTROL_SUPERVISOR.sobrecarga', '0'; '17', 'm_container', '4', '|var|CODESYS Control Win V3 x64.CONTROL_SUPERVISOR.m_container', '0'; '18', 'TLK', '4', '|var|CODESYS Control Win V3 x64.CONTROL_SUPERVISOR.TLK', '0'; '19', 'BRK_h_N1', '4', '|var|CODESYS Control Win V3 x64.CONTROL_SUPERVISOR.BRK_h_N1', '0'; '20', 'BRK_t_N1', '4', '|var|CODESYS Control Win V3 x64.CONTROL_SUPERVISOR.BRK_t_N1', '0'; '21', 'recup_ok', '4', '|var|CODESYS Control Win V3 x64.CONTROL_SUPERVISOR.recup_ok', '0'; '22', 'envolvente', '4', '|var|CODESYS Control Win V3 x64.CONTROL_SUPERVISOR.envolvente', '0'; '23', 'h_vec_output', '4', '|var|CODESYS Control Win V3 x64.CONTROL_SUPERVISOR.h_vec_output', '0'; '24', 'seleccionando', '4', '|var|CODESYS Control Win V3 x64.CONTROL_SUPERVISOR.seleccionando', '0'; '25', 'error_der', '4', '|var|CODESYS Control Win V3 x64.CONTROL_SUPERVISOR.error_der', '0'; '26', 'error_inf', '4', '|var|CODESYS Control Win V3 x64.CONTROL_SUPERVISOR.error_inf', '0'; '27', 'error_izq', '4', '|var|CODESYS Control Win V3 x64.CONTROL_SUPERVISOR.error_izq', '0'; '28', 'error_sup', '4', '|var|CODESYS Control Win V3 x64.CONTROL_SUPERVISOR.error_sup', '0' }  ShowQualityPort=off  ShowTimestampPort=off  ShowTimestampPortAs=Seconds since start  SampleTime=0.5
  SUPERVISOR OPC UA Write : opcualib/OPC UA Write  Commented=on  SelectedServer=OPCUAServer@Nahuel  ServerList=OPCUAServer@Nahuel  SampleTime=0.5  NodeList={ '1', 'Joy_XY', '4', '|var|CODESYS Control Win V3 x64.CONTROL_SUPERVISOR.Joy_XY', '0'; '2', 'BTN_TLK', '4', '|var|CODESYS Control Win V3 x64.CONTROL_SUPERVISOR.BTN_TLK', '0'; '3', 'BTN_Manual', '4', '|var|CODESYS Control Win V3 x64.CONTROL_SUPERVISOR.BTN_Manual', '0'; '4', 'BTN_Auto', '4', '|var|CODESYS Control Win V3 x64.CONTROL_SUPERVISOR.BTN_Auto', '0'; '5', 'BTN_Reset', '4', '|var|CODESYS Control Win V3 x64.CONTROL_SUPERVISOR.BTN_Reset', '0'; '6', 'FC_der', '4', '|var|CODESYS Control Win V3 x64.CONTROL_SUPERVISOR.FC_der', '0'; '7', 'FC_izq', '4', '|var|CODESYS Control Win V3 x64.CONTROL_SUPERVISOR.FC_izq', '0'; '8', 'FC_sup', '4', '|var|CODESYS Control Win V3 x64.CONTROL_SUPERVISOR.FC_sup', '0'; '9', 'FC_inf', '4', '|var|CODESYS Control Win V3 x64.CONTROL_SUPERVISOR.FC_inf', '0'; '10', 'Fhw', '4', '|var|CODESYS Control Win V3 x64.CONTROL_SUPERVISOR.Fhw', '0'; '11', 'xt_enc', '4', '|var|CODESYS Control Win V3 x64.CONTROL_SUPERVISOR.xt_enc', '0'; '12', 'yh_enc', '4', '|var|CODESYS Control Win V3 x64.CONTROL_SUPERVISOR.yh_enc', '0'; '13', 'vt_obs', '4', '|var|CODESYS Control Win V3 x64.CONTROL_SUPERVISOR.vt_obs', '0'; '14', 'vh_obs', '4', '|var|CODESYS Control Win V3 x64.CONTROL_SUPERVISOR.vh_obs', '0'; '15', 'theta_l', '4', '|var|CODESYS Control Win V3 x64.CONTROL_SUPERVISOR.theta_l', '0'; '16', 'theta_l_dot', '4', '|var|CODESYS Control Win V3 x64.CONTROL_SUPERVISOR.theta_l_dot', '0'; '17', 'FALLA_H_INF', '4', '|var|CODESYS Control Win V3 x64.CONTROL_SUPERVISOR.FALLA_H_INF', '0'; '18', 'FALLA_H_SUP', '4', '|var|CODESYS Control Win V3 x64.CONTROL_SUPERVISOR.FALLA_H_SUP', '0'; '19', 'FALLA_H_SV', '4', '|var|CODESYS Control Win V3 x64.CONTROL_SUPERVISOR.FALLA_H_SV', '0'; '20', 'FALLA_MAN', '4', '|var|CODESYS Control Win V3 x64.CONTROL_SUPERVISOR.FALLA_MAN', '0'; '21', 'FALLA_T_DER', '4', '|var|CODESYS Control Win V3 x64.CONTROL_SUPERVISOR.FALLA_T_DER', '0'; '22', 'FALLA_T_IZQ', '4', '|var|CODESYS Control Win V3 x64.CONTROL_SUPERVISOR.FALLA_T_IZQ', '0'; '23', 'FALLA_WD', '4', '|var|CODESYS Control Win V3 x64.CONTROL_SUPERVISOR.FALLA_WD', '0' }
  Zero-Order Hold{33..36,38,57..74} (23 alike) : ZeroOrderHold  Commented=on  SampleTime=Ts1
  wires:
  Bus Selector1/23 -> Goto5/1  "<h_vec_output_varCODESYSControlWinV3X64CONTROL_SUPERVISORh_vec_output>"
  Bus Selector1/4 -> Goto102/1  "<vy_cmd_varCODESYSControlWinV3X64CONTROL_SUPERVISORvy_cmd>"
  From120/1 -> Zero-Order Hold70/1
  From124/1 -> Zero-Order Hold58/1
  Bus Selector1/21 -> Goto101/1  "<recup_ok_varCODESYSControlWinV3X64CONTROL_SUPERVISORrecup_ok>"
  From116/1 -> Zero-Order Hold67/1
  Bus Selector1/10 -> Cast To Single4/1  "<modo_auto_varCODESYSControlWinV3X64CONTROL_SUPERVISORmodo_auto>"
  From117/1 -> Zero-Order Hold73/1
  Bus Selector1/5 -> Cast To Single14/1  "<seleccionando_i_varCODESYSControlWinV3X64CONTROL_SUPERVISORseleccionando_i>"
  From93/1 -> Zero-Order Hold38/1
  Zero-Order Hold68/1 -> Delay One Step21/1
  SUPERVISOR OPC UA Read/1 -> Bus Selector1/1
  Cast To Single/1 -> Goto83/1
  Zero-Order Hold61/1 -> SUPERVISOR OPC UA Write/4
  Zero-Order Hold71/1 -> SUPERVISOR OPC UA Write/18
  Zero-Order Hold59/1 -> SUPERVISOR OPC UA Write/8
  Bus Selector1/18 -> Cast To Single12/1  "<TLK_varCODESYSControlWinV3X64CONTROL_SUPERVISORTLK>"
  Zero-Order Hold58/1 -> Delay One Step25/1
  Delay One Step22/1 -> SUPERVISOR OPC UA Write/15
  Zero-Order Hold63/1 -> SUPERVISOR OPC UA Write/7
  Bus Selector1/27 -> Cast To Single21/1  "<error_izq_varCODESYSControlWinV3X64CONTROL_SUPERVISORerror_izq>"
  Cast To Single20/1 -> Goto46/1
  From123/1 -> Zero-Order Hold74/1
  Bus Selector1/20 -> Goto90/1  "<BRK_t_N1_varCODESYSControlWinV3X64CONTROL_SUPERVISORBRK_t_N1>"
  Cast To Single21/1 -> Goto48/1
  Cast To Single18/1 -> Goto45/1
  Bus Selector1/28 -> Cast To Single22/1  "<error_sup_varCODESYSControlWinV3X64CONTROL_SUPERVISORerror_sup>"
  Bus Selector1/8 -> Goto86/1  "<y_cruz_unity_varCODESYSControlWinV3X64CONTROL_SUPERVISORy_cruz_unity>"
  Cast To Single12/1 -> Goto80/1
  Cast To Single4/1 -> Goto82/1
  Zero-Order Hold62/1 -> Delay One Step26/1
  Bus Selector1/25 -> Cast To Single19/1  "<error_der_varCODESYSControlWinV3X64CONTROL_SUPERVISORerror_der>"
  Bus Selector1/15 -> Cast To Single1/1  "<ejec_mov_varCODESYSControlWinV3X64CONTROL_SUPERVISORejec_mov>"
  Cast To Single5/1 -> Goto95/1
  Bus Selector1/13 -> Cast To Single7/1  "<modo_manual_auto_varCODESYSControlWinV3X64CONTROL_SUPERVISORmodo_manual_auto>"
  From118/1 -> Zero-Order Hold62/1
  Delay One Step23/1 -> SUPERVISOR OPC UA Write/16
  From122/1 -> Zero-Order Hold66/1
  Zero-Order Hold57/1 -> SUPERVISOR OPC UA Write/6
  Delay One Step20/1 -> SUPERVISOR OPC UA Write/11
  Bus Selector1/1 -> Goto79/1  "<m_est_varCODESYSControlWinV3X64CONTROL_SUPERVISORm_est>"
  OPC UA Read1/1 -> Goto100/1
  From119/1 -> Zero-Order Hold65/1
  Bus Selector1/9 -> Cast To Single3/1  "<modo_manual_varCODESYSControlWinV3X64CONTROL_SUPERVISORmodo_manual>"
  Bus Selector1/26 -> Cast To Single20/1  "<error_inf_varCODESYSControlWinV3X64CONTROL_SUPERVISORerror_inf>"
  Zero-Order Hold69/1 -> SUPERVISOR OPC UA Write/1
  Cast To Single22/1 -> Goto47/1
  From79/1 -> Zero-Order Hold72/1
  Delay One Step26/1 -> SUPERVISOR OPC UA Write/13
  Zero-Order Hold73/1 -> Delay One Step23/1
  Cast To Single3/1 -> Goto81/1
  From121/1 -> Zero-Order Hold60/1
  Zero-Order Hold74/1 -> SUPERVISOR OPC UA Write/5
  Zero-Order Hold34/1 -> SUPERVISOR OPC UA Write/20
  Cast To Single1/1 -> Goto99/1
  From59/1 -> Zero-Order Hold36/1
  Cast To Single6/1 -> Goto96/1
  From126/1 -> Zero-Order Hold69/1
  Zero-Order Hold64/1 -> SUPERVISOR OPC UA Write/9
  Bus Selector1/7 -> Goto87/1  "<x_cruz_unity_varCODESYSControlWinV3X64CONTROL_SUPERVISORx_cruz_unity>"
  Cast To Single2/1 -> Goto98/1
  Zero-Order Hold72/1 -> SUPERVISOR OPC UA Write/17
  Bus Selector1/14 -> Cast To Single2/1  "<modo_standby_varCODESYSControlWinV3X64CONTROL_SUPERVISORmodo_standby>"
  Bus Selector1/12 -> Cast To Single6/1  "<modo_error_varCODESYSControlWinV3X64CONTROL_SUPERVISORmodo_error>"
  Bus Selector1/3 -> Goto84/1  "<vx_cmd_varCODESYSControlWinV3X64CONTROL_SUPERVISORvx_cmd>"
  Cast To Single14/1 -> Goto88/1
  From131/1 -> Zero-Order Hold57/1
  Bus Selector1/17 -> Goto85/1  "<m_container_varCODESYSControlWinV3X64CONTROL_SUPERVISORm_container>"
  From129/1 -> Zero-Order Hold59/1
  From125/1 -> Zero-Order Hold61/1
  Cast To Single19/1 -> Goto49/1
  From130/1 -> Zero-Order Hold63/1
  Zero-Order Hold36/1 -> SUPERVISOR OPC UA Write/21
  Zero-Order Hold35/1 -> SUPERVISOR OPC UA Write/22
  From74/1 -> Zero-Order Hold33/1
  From80/1 -> Zero-Order Hold34/1
  Delay One Step24/1 -> SUPERVISOR OPC UA Write/14
  From75/1 -> Zero-Order Hold71/1
  Cast To Single7/1 -> Goto97/1
  Delay One Step21/1 -> SUPERVISOR OPC UA Write/12
  Delay One Step25/1 -> SUPERVISOR OPC UA Write/10
  Zero-Order Hold65/1 -> Delay One Step22/1
  From128/1 -> Zero-Order Hold68/1
  Zero-Order Hold66/1 -> SUPERVISOR OPC UA Write/3
  Cast To Single13/1 -> Goto94/1
  Zero-Order Hold33/1 -> SUPERVISOR OPC UA Write/19
  Bus Selector1/2 -> Goto78/1  "<vh_lim_varCODESYSControlWinV3X64CONTROL_SUPERVISORvh_lim>"
  Bus Selector1/19 -> Goto89/1  "<BRK_h_N1_varCODESYSControlWinV3X64CONTROL_SUPERVISORBRK_h_N1>"
  Bus Selector1/24 -> Cast To Single18/1  "<seleccionando_varCODESYSControlWinV3X64CONTROL_SUPERVISORseleccionando>"
  Zero-Order Hold60/1 -> SUPERVISOR OPC UA Write/2
  Bus Selector1/11 -> Cast To Single5/1  "<modo_posicion_segura_varCODESYSControlWinV3X64CONTROL_SUPERVISORmodo_posicion_segura>"
  From127/1 -> Zero-Order Hold64/1
  Zero-Order Hold38/1 -> SUPERVISOR OPC UA Write/23
  Zero-Order Hold67/1 -> Delay One Step20/1
  Bus Selector1/16 -> Cast To Single/1  "<sobrecarga_varCODESYSControlWinV3X64CONTROL_SUPERVISORsobrecarga>"
  Zero-Order Hold70/1 -> Delay One Step24/1
  Bus Selector1/22 -> Goto91/1  "<envolvente_varCODESYSControlWinV3X64CONTROL_SUPERVISORenvolvente>"
  Bus Selector1/6 -> Cast To Single13/1  "<i_obj_vec_varCODESYSControlWinV3X64CONTROL_SUPERVISORi_obj_vec>"
  From10/1 -> Zero-Order Hold35/1

== system planta_CODESYS/Controlador Carro2 ==
  xtd_enc : Inport
  θ_l : Inport  Port=2
  vx_cmd : Inport  Port=3
  BRK_t : Inport  Port=4
  anti-sway : Inport  Port=5
  seleccion : Inport  Port=6
  yh_enc : Inport  Port=7
  Controlador de Balanceo : MATLAB Function  TreatAsAtomicUnit=on
  Controlador de Velocidad : MATLAB Function  TreatAsAtomicUnit=on
  Delay : Delay  DelayLength=1  InitialCondition=Ttm_0
  Modulación de la Referencia : MATLAB Function  TreatAsAtomicUnit=on
  Observador de Estado : MATLAB Function  TreatAsAtomicUnit=on
  Ttm_ref : Outport
  vt_obs : Outport  Port=2
  wires:
  seleccion/1 -> Modulación de la Referencia/2(seleccion)
  θ_l/1 -> Controlador de Balanceo/1(tita_l)
  vx_cmd/1 -> Modulación de la Referencia/1(vx_cmd)
  yh_enc/1 -> Controlador de Balanceo/2(yh_enc)
  Controlador de Balanceo/1(v_sway) -> Modulación de la Referencia/3(v_sway)
  Observador de Estado/1(vt_obs) -> vt_obs/1, Controlador de Velocidad/2(vt_obs)
  BRK_t/1 -> Controlador de Velocidad/3(BRK_t)
  Delay/1 -> Observador de Estado/2(Ttm_ref)
  xtd_enc/1 -> Observador de Estado/1(xtd_enc)
  Modulación de la Referencia/1(vt_ref) -> Controlador de Velocidad/1(vt_ref)
  anti-sway/1 -> Controlador de Balanceo/3(anti_sway)
  Controlador de Velocidad/1(Ttm_ref) -> Delay/1, Ttm_ref/1
